simulink model "rotpentemplateV6"  (R2025a)
settings: Solver=ode45  StartTime=0.0  StopTime=run_time  RelTol=1e-3  EnableMultiTasking=on
values from neighbouring files (symbols this model uses):
  A = 0.2    [Multisine_test.m]    (also in compute_lqr.m = double(subs(subs(A_sym, x, x0), u, 0)); compute_mpc.m = double(subs(subs(A_sym, x, x0), u, 0)); link2_ode.m = [0 1; -beta -alpha]; my_pendulum_model.m = [0,  1,  0,  0)
  adingain = [adingain 1 1 1 1 1]    [hwinit.m]
  adinoffs = [adinoffs 0 0 0 0 0]    [hwinit.m]
  B = zeros(n, nu)    [Multisine_test.m]    (also in compute_lqr.m = double(subs(subs(B_sym, x, x0), u, 0)); compute_mpc.m = double(subs(subs(B_sym, x, x0), u, 0)); link2_ode.m = zeros(2, 0); my_pendulum_model.m = [0; b; 0; 0])
  C = [1 0 0 0 ... (first row only)    [Multisine_test.m]    (also in compute_lqr.m; compute_mpc.m; link2_ode.m = [1 0]; my_pendulum_model.m = eye(4))
  controller_sat = 1    [run_controller.m]    (also in run_freeswing.m = 0; run_lqr.m; run_mpc.m; run_ref_tracking.m)
  daoutgain = 1*[-6]    [hwinit.m]
  daoutoffs = [0.00]    [hwinit.m]
  h = 0.01    [Multisine_test.m]    (also in animate_pendulum.m = mean(diff(t)); collect_arm2_freeswing.m; collect_freeswing.m; first-script.m)
  K = lqr(A, B, Q, R)    [compute_lqr.m]    (also in link2_ode.m = zeros(2, 1); run_controller.m = K_full; run_ref_tracking.m = K_full(1:4))
  L = [31.5412926965  -1.46586450973  1.48832994181  104.88438352; 1.48832994181  0.281132012302  39.1187891696  266.247396057]    [lqr_gains.mat]
  offset = [pi; 0]    [run_controller.m]    (also in run_lqr.m; run_mpc.m; run_ref_tracking.m = [0; -pi])
  ref = [-pi; 0; 0; 0]    [run_controller.m]    (also in run_lqr.m = [pi; 0; 0; 0]; run_mpc.m = [pi; 0]; run_ref_tracking.m = ref_eq)
undefined symbols (not defined in the file or in its folder): A_d, A_k, eps_v, f_d, f_k, jiggle_mode, tau_lp, u_min
libraries: simulink_extras x1
settings Model: Creator=rbabuska  LastModifiedBy=thomas
settings SolverCC: AlgebraicLoopSolver=TrustRegion
settings DataIOCC: SaveFormat=Array  ReturnWorkspaceOutputs=off  SignalLoggingName=sigsOut
settings OptimizationCC: BooleanDataType=off  ExpressionDepthLimit=2147483647.0  InitFltsAndDblsToZero=on  LifeSpan=inf
settings DebuggingCC: SaveWithParameterizedLinksMsg=none  SignalResolutionControl=TryResolveAllWithWarning  MultiTaskDSMMsg=warning  MultiTaskCondExecSysMsg=none  UnconnectedInputMsg=warning  UnconnectedOutputMsg=warning  UnconnectedLineMsg=warning  AllowSymbolicDim=off  StateNameClashWarn=warning  SFUnexpectedBacktrackingDiag=warning  SFNoUnconditionalDefaultTransitionDiag=warning  SFExecutionAtInitializationDiag=none  ArithmeticOperatorsInVariantConditions=warning
settings HardwareCC: ProdBitPerPointer=32.0  ProdBitPerSizeT=32.0  ProdBitPerPtrDiffT=32.0  ProdLargestAtomicFloat=None  ProdIntDivRoundTo=Undefined  ProdEndianess=Unspecified  ProdWordSize=32.0  ProdHWDeviceType=32-bit Generic  TargetUnknown=on
settings ModelReferenceCC: EnableRefExpFcnMdlSchedulingChecks=on  PropagateSignalLabelsOutOfModel=off
settings SFSimCC: SimUseLocalCustomCode=off  CustomCodeUndefinedFunction=UseInterfaceOnly
settings RTWCC: RTWUseLocalCustomCode=off  GPUComputeCapability=3.5  DLArmComputeVersion=19.05
settings CodeAppCC: StateflowObjectComments=on
settings GRTTargetCC: TargetFcnLib=ansi_tfl_tmw.mat  TargetLangStandard=C89/C90 (ANSI)  CombineOutputUpdateFcns=off  GRTInterface=on
settings ConfigComp: CovMetricSettings=dw  CovSaveCumulativeToWorkspaceVar=on  CovSaveSingleToWorkspaceVar=on  CovExternalEMLEnable=off

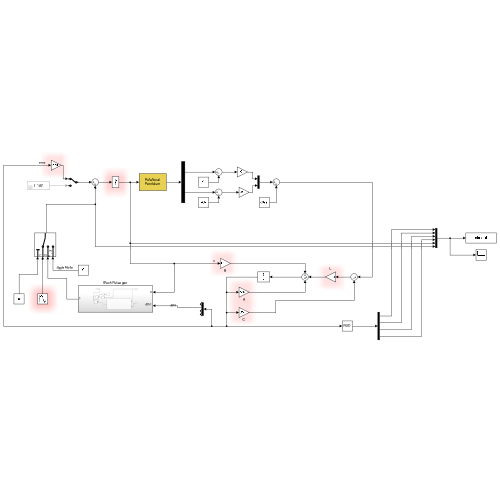
[thumbnail: Simulink's stored preview of the top-level diagram]
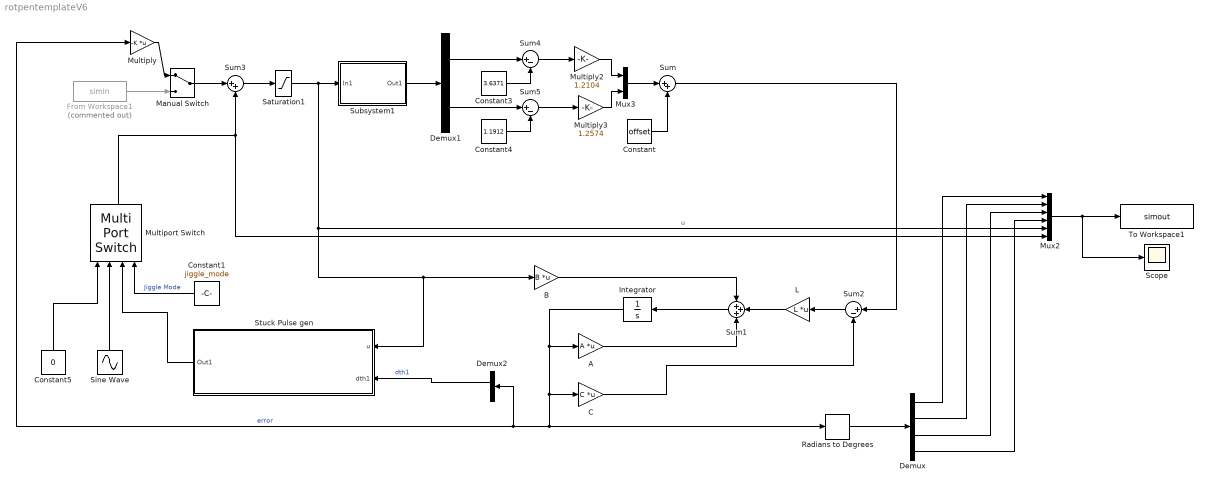
== system rotpentemplateV6 ==
  A : Gain  Gain=A  Multiplication=Matrix(K*u)
  B : Gain  Gain=B  Multiplication=Matrix(K*u)
  C : Gain  Gain=C  Multiplication=Matrix(K*u)
  Constant : Constant  Value=offset
  Constant1 : Constant  Value=jiggle_mode
  Constant3 : Constant  Value=3.6371
  Constant4 : Constant  Value=1.1912
  Constant5 : Constant  Value=0
  Demux : Demux
  Demux1 : Demux  Outputs=2
  Demux2 : Demux
  From Workspace1 : FromWorkspace  Commented=on  VariableName=simin
  Integrator : Integrator  InitialCondition=0*ref
  L : Gain  Gain=L  Multiplication=Matrix(K*u)
  Manual Switch : ManualSwitch
  Multiply : Gain  Gain=-K  Multiplication=Matrix(K*u)
  Multiply2 : Gain  Gain=1.2104
  Multiply3 : Gain  Gain=1.2574
  Multiport Switch : MultiPortSwitch  SaturateOnIntegerOverflow=off  InputSameDT=off
  Mux2 : Mux  Inputs=6
  Mux3 : Mux  Inputs=2
  Radians to Degrees : simulink_extras/Transformations/Radians to Degrees
  Saturation1 : Saturate  UpperLimit=controller_sat  LowerLimit=-controller_sat
  Scope : Scope
  Sine Wave : Sin  Amplitude=A_d  Frequency=f_d  SampleTime=h
  Stuck Pulse gen : Subsystem
  Subsystem1 : Subsystem
      mask Display: disp('Rotational\nPendulum')
  Sum : Sum  Inputs=|++
  Sum1 : Sum  Inputs=+++
  Sum2 : Sum  Inputs=|+-
  Sum3 : Sum  Inputs=|++
  Sum4 : Sum  Inputs=|+-
  Sum5 : Sum  Inputs=|+-
  To Workspace1 : ToWorkspace  VariableName=simout  SaveFormat=Timeseries  SampleTime=-1
  wires:
  Constant3/1 -> Sum4/2
  Mux2/1 -> To Workspace1/1, Scope/1
  Sum5/1 -> Multiply3/1
  Sum4/1 -> Multiply2/1
  Demux1/1 -> Sum4/1
  Constant4/1 -> Sum5/2
  Demux1/2 -> Sum5/1
  Saturation1/1 -> Stuck Pulse gen/1(u), B/1, Mux2/5, Subsystem1/1(In1)  "u"
  Subsystem1/1(Out1) -> Demux1/1
  Integrator/1 -> A/1, Demux2/1, Multiply/1, Radians to Degrees/1, C/1  "error"
  From Workspace1/1 -> Manual Switch/2
  B/1 -> Sum1/1
  Sum1/1 -> Integrator/1
  A/1 -> Sum1/3
  L/1 -> Sum1/2
  Demux/1 -> Mux2/1
  Demux/2 -> Mux2/2
  Demux/3 -> Mux2/3
  Demux/4 -> Mux2/4
  Multiply/1 -> Manual Switch/1
  Sum2/1 -> L/1
  C/1 -> Sum2/2
  Radians to Degrees/1 -> Demux/1
  Multiply2/1 -> Mux3/1
  Multiply3/1 -> Mux3/2
  Mux3/1 -> Sum/1
  Constant/1 -> Sum/2
  Sum/1 -> Sum2/1
  Constant5/1 -> Multiport Switch/1
  Sine Wave/1 -> Multiport Switch/2
  Demux2/2 -> Stuck Pulse gen/2(dth1)  "dth1"
  Stuck Pulse gen/1(Out1) -> Multiport Switch/3
  Constant1/1 -> Multiport Switch/4  "Jiggle Mode"
  Manual Switch/1 -> Sum3/1
  Sum3/1 -> Saturation1/1
  Multiport Switch/1 -> Mux2/6, Sum3/2

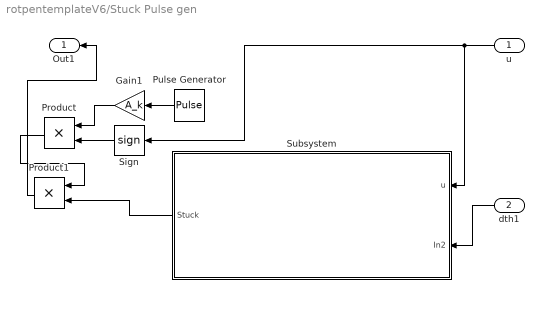
== system rotpentemplateV6/Stuck Pulse gen ==
  u : Inport
  dth1 : Inport  Port=2
  Gain1 : Gain  Gain=A_k
  Product : Product
  Product1 : Product
  Pulse Generator : DiscretePulseGenerator  PulseType=Time based  Period=1/f_k  PulseWidth=50
  Sign : Signum
  Subsystem : Subsystem
  Out1 : Outport
  wires:
  u/1 -> Subsystem/1(u), Sign/1
  Pulse Generator/1 -> Gain1/1
  Subsystem/1(Stuck) -> Product1/2
  dth1/1 -> Subsystem/2(In2)
  Product1/1 -> Out1/1
  Sign/1 -> Product/2
  Gain1/1 -> Product/1
  Product/1 -> Product1/1

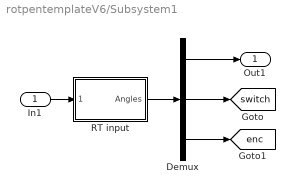
== system rotpentemplateV6/Subsystem1 ==
  In1 : Inport
  Demux : Demux  Outputs=[2 4 1]
  RT input : Subsystem  mask{Ts=h, channels=[6 7]}
      mask prompts: Ts "Sample time [s]:"; channels "Channels to read (e.g., [6 7])"
      mask init:
      | hwinit;
      | 
      | % initialize FPGA
      | fugihandle = fugiboard('Open', 'Pendulum1');
      | fugihandle.WatchdogTimeout = 0.5;
      | fugiboard('SetParams', fugihandle);
      | fugiboard('Write', fugihandle, 0, 0, 0, 0);  % dummy write to sync interface board
      | fugiboard('Write', fugihandle, 5, 1, 0, 0);  % reset position, activate relay
      | data = fugiboard('Read', fugihandle);        % get version info from FPGA
      | % model = bitshift(data(1), -5); 
      | % version = bitand(data(1), 31);
      | % disp(sprintf('FPGA setup %d, version %d', model, version)); % for the B&P it should say 1 1, or else there is a problem
      | fugiboard('Write', fugihandle, 0, 1, 0, 0);  % end reset
      | pause(0.1);                         % give relay some time to respond
      mask Display: disp('Rotational\nPendulum')
  Out1 : Outport
  tag scope: enc=global, switch=global
  wires:
  RT input/1(Angles) -> Demux/1
  Demux/1 -> Out1/1
  In1/1 -> RT input/1(Motors)
  Demux/2 -> [switch]
  Demux/3 -> [enc]

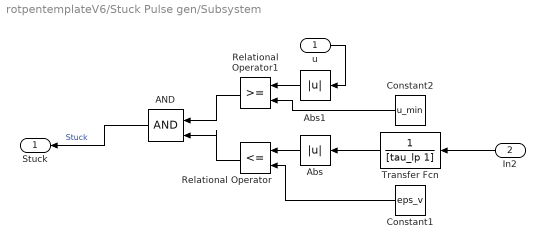
== system rotpentemplateV6/Stuck Pulse gen/Subsystem ==
  u : Inport
  In2 : Inport  Port=2
  AND : Logic  IconShape=distinctive  AllPortsSameDT=off  OutDataTypeStr=boolean
  Abs : Abs  SaturateOnIntegerOverflow=off
  Abs1 : Abs  SaturateOnIntegerOverflow=off
  Constant1 : Constant  Value=eps_v
  Constant2 : Constant  Value=u_min
  Relational Operator : RelationalOperator  Operator=<=  OutDataTypeStr=boolean  RndMeth=Simplest  InputSameDT=off
  Relational Operator1 : RelationalOperator  OutDataTypeStr=boolean  RndMeth=Simplest  InputSameDT=off
  Transfer Fcn : TransferFcn  Denominator=[tau_lp 1]  ContinuousStateAttributes='dth1'
  Stuck : Outport
  wires:
  AND/1 -> Stuck/1  "Stuck"
  Relational Operator/1 -> AND/2
  Constant1/1 -> Relational Operator/2
  u/1 -> Abs1/1
  Constant2/1 -> Relational Operator1/2
  Relational Operator1/1 -> AND/1
  Transfer Fcn/1 -> Abs/1
  Abs/1 -> Relational Operator/1
  In2/1 -> Transfer Fcn/1
  Abs1/1 -> Relational Operator1/1

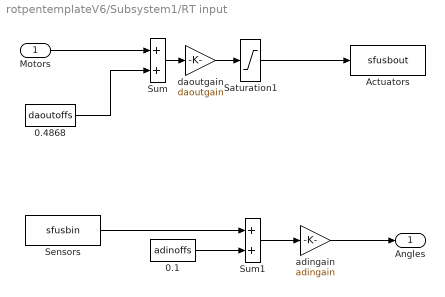
== system rotpentemplateV6/Subsystem1/RT input ==
  Motors : Inport
  0.1 : Constant  Value=adinoffs
  0.4868 : Constant  Value=daoutoffs
  Actuators : S-Function  FunctionName=sfusbout  Parameters=Ts, fugihandle  SFunctionDeploymentMode=off  EnableBusSupport=off
  Saturation1 : Saturate  UpperLimit=10  LowerLimit=-10
  Sensors : S-Function  FunctionName=sfusbin  Parameters=Ts, fugihandle, channels  SFunctionDeploymentMode=off  EnableBusSupport=off
  Sum : Sum  InputSameDT=on  SaturateOnIntegerOverflow=on  OutDataTypeStr=Inherit: Same as first input
  Sum1 : Sum  InputSameDT=on  SaturateOnIntegerOverflow=on  OutDataTypeStr=Inherit: Same as first input
  adingain : Gain  Gain=adingain  SaturateOnIntegerOverflow=on  OutDataTypeStr=Inherit: Same as input  ParamDataTypeStr=Inherit: Same as input
  daoutgain : Gain  Gain=daoutgain  SaturateOnIntegerOverflow=on  OutDataTypeStr=Inherit: Same as input  ParamDataTypeStr=Inherit: Same as input
  Angles : Outport
  wires:
  Sum/1 -> daoutgain/1
  0.4868/1 -> Sum/2
  Motors/1 -> Sum/1
  Sum1/1 -> adingain/1
  0.1/1 -> Sum1/2
  adingain/1 -> Angles/1
  Saturation1/1 -> Actuators/1
  daoutgain/1 -> Saturation1/1
  Sensors/1 -> Sum1/1
